simulink model "Pendulum"  (R2024b)
settings: Solver=FixedStepAuto  StartTime=0.0  StopTime=inf  RelTol=1e-3
libraries: slrealtimeethercatlib x13, simulink x2
settings Model: Creator=Wave User  LastModifiedBy=Wave User
settings SolverCC: ConcurrentTasks=on  PositivePriorityOrder=on
settings OptimizationCC: BlockReduction=off  OptimizeBlockIOStorage=off
settings DebuggingCC: TasksWithSamePriorityMsg=none
settings HardwareCC: ProdBitPerLong=64  ProdLongLongMode=on  ProdHWDeviceType=Intel->x86-64 (Linux 64)
settings RTWCC: Description=Speedgoat Real-Time Target Machine  SystemTargetFile=speedgoat.tlc  TemplateMakefile=slrealtime_default_tmf  Toolchain=Simulink Real-Time Toolchain  BuildConfiguration=Faster Runs  CodeExecutionProfiling=on  TargetLang=C++
settings SimulinkRealTimeTargetCC: InstructionSetFMA=off  LogToMDFFile=off

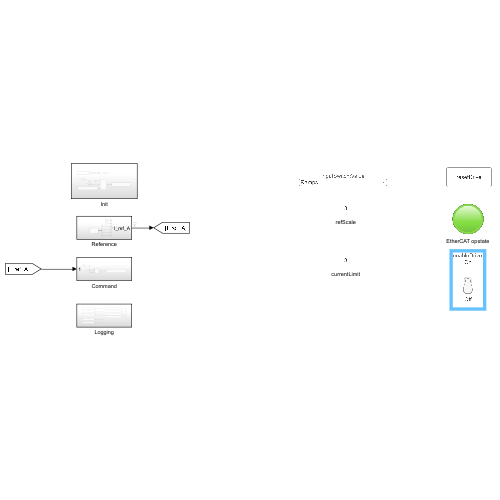
[thumbnail: Simulink's stored preview of the top-level diagram]
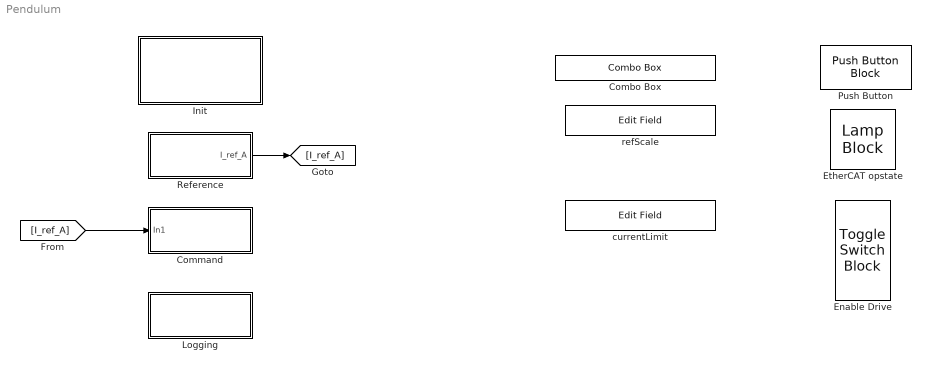
== system Pendulum ==
  Combo Box : ComboBox  SelectedLabel=Ramps
      settings: Values={{'Ramps', 'Sine', 'Chirp', 'BLWN', 'None'}, [2 3 4 5 1]}
  Command : Subsystem
  Enable Drive : ToggleSwitchBlock
      settings: Values={{'Off', 'On'}, [0 1]}
  EtherCAT opstate : LampBlock  LabelPosition=Hide
  Init : Subsystem
  Logging : Subsystem
  Push Button : PushButtonBlock  ButtonText=resetDrive  OffValue=0.000000
  Reference : Subsystem
  currentLimit : EditField  LabelPosition=Hide  ShowInitialText=on  Alignment=Center
  refScale : EditField  LabelPosition=Hide  ShowInitialText=on  Alignment=Center
  wires:
  Reference/1(I_ref_A) -> [I_ref_A]
  [I_ref_A] -> Command/1(In1)

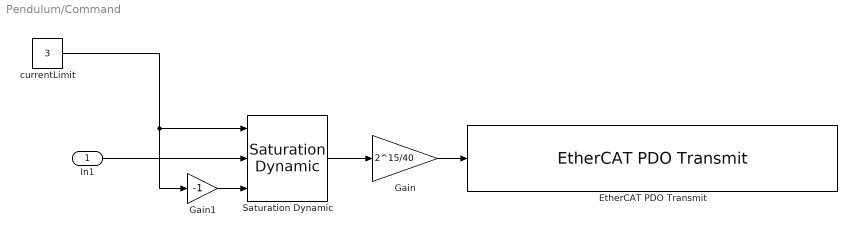
== system Pendulum/Command ==
  In1 : Inport
  EtherCAT PDO Transmit : slrealtimeethercatlib/EtherCAT PDO Transmit  Priority=3  sig_name=Drive 6 (AMC).Module 1 (Default).PDO data to Slave.Target Current  sig_offset=696  sig_type=int16  type_size=16  sig_dim=1  device_id=0  sample_time=0.001000
  Gain : Gain  Gain=2^15/40  OutDataTypeStr=int16
  Gain1 : Gain  Gain=-1
  Saturation Dynamic : simulink/Discontinuities/Saturation Dynamic  OutMin=[]  OutMax=[]  OutDataTypeStr=Inherit: Same as second input  OutDataType=fixdt(1, 16)  OutScaling=2^-10  DoSatur=off
  currentLimit : Constant  Value=3  OutDataTypeStr=Inherit: Inherit via back propagation
  wires:
  Saturation Dynamic/1 -> Gain/1
  Gain/1 -> EtherCAT PDO Transmit/1
  In1/1 -> Saturation Dynamic/2
  currentLimit/1 -> Gain1/1, Saturation Dynamic/1
  Gain1/1 -> Saturation Dynamic/3

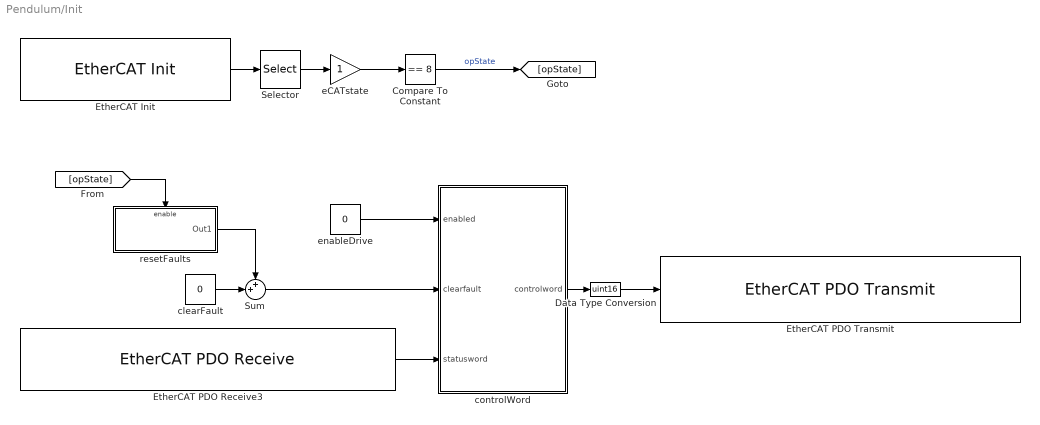
== system Pendulum/Init ==
  Compare To Constant : simulink/Logic and Bit Operations/Compare To Constant  relop===  const=8  OutDataTypeStr=boolean
  Data Type Conversion : DataTypeConversion  OutDataTypeStr=uint16  SaturateOnIntegerOverflow=off  RndMeth=Floor
  EtherCAT Init : slrealtimeethercatlib/EtherCAT Init  Priority=0  config_file=C:\Software\WEC-Bench\TwinCAT3\Pendulum2XML.xml  device_id=0  portnum=1  initstate=2  dctuning=0  enaDebug=0  logFile='c:\dbglog.txt'  sample_time=0.001000  DCMode=2
  EtherCAT PDO Receive3 : slrealtimeethercatlib/EtherCAT PDO Receive  Priority=2  sig_name=Drive 6 (AMC).Module 1 (Default).PDO data from Slave.Status Word  sig_offset=616  sig_type=uint16  type_size=16  sig_dim=1  device_id=0  sample_time=0.001000
  EtherCAT PDO Transmit : slrealtimeethercatlib/EtherCAT PDO Transmit  Priority=3  sig_name=Drive 6 (AMC).Module 1 (Default).PDO data to Slave.Control Word  sig_offset=616  sig_type=uint16  type_size=16  sig_dim=1  device_id=0  sample_time=0.001000
  Selector : Selector  InputPortWidth=6  IndexOptions=Index vector (dialog)  Indices=2  OutputSizes=1
  Sum : Sum  Inputs=++|
  clearFault : Constant  Value=0  OutDataTypeStr=Inherit: Inherit via back propagation
  controlWord : MATLAB Function  TreatAsAtomicUnit=on
  eCATstate : Gain  OutDataTypeStr=double
  enableDrive : Constant  Value=0
  resetFaults : Subsystem  TreatAsAtomicUnit=on
  wires:
  EtherCAT Init/1 -> Selector/1
  EtherCAT PDO Receive3/1 -> controlWord/3(statusword)
  eCATstate/1 -> Compare To Constant/1
  controlWord/1(controlword) -> Data Type Conversion/1
  Compare To Constant/1 -> [opState]  "opState"
  Selector/1 -> eCATstate/1
  enableDrive/1 -> controlWord/1(enabled)
  Sum/1 -> controlWord/2(clearfault)
  clearFault/1 -> Sum/2
  [opState] -> resetFaults/Enable
  resetFaults/1(Out1) -> Sum/1
  Data Type Conversion/1 -> EtherCAT PDO Transmit/1

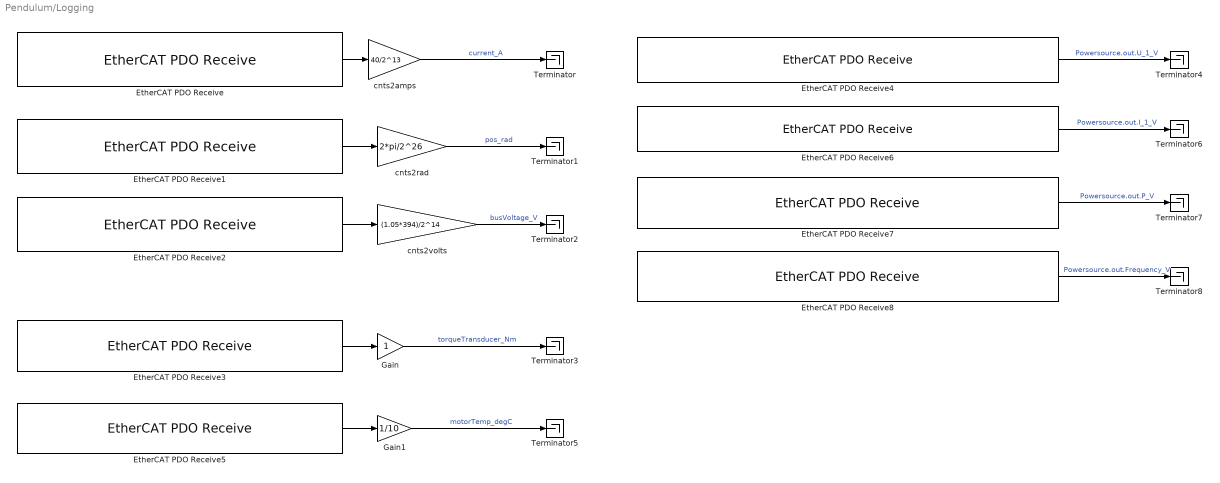
== system Pendulum/Logging ==
  EtherCAT PDO Receive : slrealtimeethercatlib/EtherCAT PDO Receive  Priority=2  sig_name=Drive 6 (AMC).Module 1 (Default).PDO data from Slave.Actual Current  sig_offset=696  sig_type=int16  type_size=16  sig_dim=1  device_id=0  sample_time=0.001000
  EtherCAT PDO Receive1 : slrealtimeethercatlib/EtherCAT PDO Receive  Priority=2  sig_name=Drive 6 (AMC).Module 1 (Default).PDO data from Slave.Actual position  sig_offset=632  sig_type=int32  type_size=32  sig_dim=1  device_id=0  sample_time=0.001000
  EtherCAT PDO Receive2 : slrealtimeethercatlib/EtherCAT PDO Receive  Priority=2  sig_name=Drive 6 (AMC).Module 1 (Default).PDO data from Slave.DC Bus Voltage  sig_offset=728  sig_type=int16  type_size=16  sig_dim=1  device_id=0  sample_time=0.001000
  EtherCAT PDO Receive3 : slrealtimeethercatlib/EtherCAT PDO Receive  Priority=2  sig_name=Term 4 (EL3356-0010).RMB Value (Real).Value (Real)  sig_offset=584  sig_type=single  type_size=32  sig_dim=1  device_id=0  sample_time=0.001000
  EtherCAT PDO Receive4 : slrealtimeethercatlib/EtherCAT PDO Receive  Priority=2  sig_name=Box 8 (GEN Series DAQ System).Powersource.out.U_1.Powersource.out.U_1_V  sig_offset=1336  sig_type=single  type_size=32  sig_dim=1  device_id=0  sample_time=0.001000
  EtherCAT PDO Receive5 : slrealtimeethercatlib/EtherCAT PDO Receive  Priority=2  sig_name=Term 5 (EL3201).RTD.Value  sig_offset=856  sig_type=int16  type_size=16  sig_dim=1  device_id=0  sample_time=0.001000
  EtherCAT PDO Receive6 : slrealtimeethercatlib/EtherCAT PDO Receive  Priority=2  sig_name=Box 8 (GEN Series DAQ System).Powersource.out.I_1.Powersource.out.I_1_V  sig_offset=1176  sig_type=single  type_size=32  sig_dim=1  device_id=0  sample_time=0.001000
  EtherCAT PDO Receive7 : slrealtimeethercatlib/EtherCAT PDO Receive  Priority=2  sig_name=Box 8 (GEN Series DAQ System).Powersource.out.P.Powersource.out.P_V  sig_offset=1616  sig_type=single  type_size=32  sig_dim=1  device_id=0  sample_time=0.001000
  EtherCAT PDO Receive8 : slrealtimeethercatlib/EtherCAT PDO Receive  Priority=2  sig_name=Box 8 (GEN Series DAQ System).Powersource.out.Frequency.Powersource.out.Frequency_V  sig_offset=1136  sig_type=single  type_size=32  sig_dim=1  device_id=0  sample_time=0.001000
  Gain : Gain  OutDataTypeStr=double
  Gain1 : Gain  Gain=1/10
  Terminator{,1..8} (9 alike) : Terminator
  cnts2amps : Gain  Gain=40/2^13  OutDataTypeStr=double
  cnts2rad : Gain  Gain=2*pi/2^26  OutDataTypeStr=double
  cnts2volts : Gain  Gain=(1.05*394)/2^14
  wires:
  EtherCAT PDO Receive/1 -> cnts2amps/1
  cnts2amps/1 -> Terminator/1  "current_A"
  EtherCAT PDO Receive1/1 -> cnts2rad/1
  cnts2rad/1 -> Terminator1/1  "pos_rad"
  EtherCAT PDO Receive2/1 -> cnts2volts/1
  cnts2volts/1 -> Terminator2/1  "busVoltage_V"
  EtherCAT PDO Receive3/1 -> Gain/1
  Gain/1 -> Terminator3/1  "torqueTransducer_Nm"
  EtherCAT PDO Receive4/1 -> Terminator4/1  "Powersource.out.U_1_V"
  EtherCAT PDO Receive5/1 -> Gain1/1
  Gain1/1 -> Terminator5/1  "motorTemp_degC"
  EtherCAT PDO Receive6/1 -> Terminator6/1  "Powersource.out.I_1_V"
  EtherCAT PDO Receive7/1 -> Terminator7/1  "Powersource.out.P_V"
  EtherCAT PDO Receive8/1 -> Terminator8/1  "Powersource.out.Frequency_V"

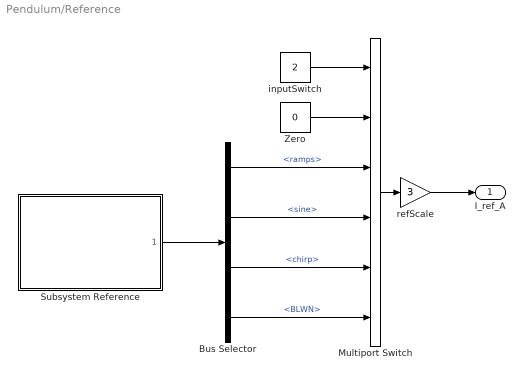
== system Pendulum/Reference ==
  Bus Selector : BusSelector  OutputSignals=ramps,sine,chirp,BLWN
  Multiport Switch : MultiPortSwitch  Inputs=5  SaturateOnIntegerOverflow=off  InputSameDT=off
  Subsystem Reference : Subsystem  ReferencedSubsystem=referenceSigs
  Zero : Constant  Value=0  OutDataTypeStr=Inherit: Inherit via back propagation
  inputSwitch : Constant  Value=2
  refScale : Gain  Gain=3
  I_ref_A : Outport
  wires:
  Subsystem Reference/1 -> Bus Selector/1
  Zero/1 -> Multiport Switch/2
  Bus Selector/1 -> Multiport Switch/3  "<ramps>"
  Bus Selector/2 -> Multiport Switch/4  "<sine>"
  Bus Selector/3 -> Multiport Switch/5  "<chirp>"
  Bus Selector/4 -> Multiport Switch/6  "<BLWN>"
  Multiport Switch/1 -> refScale/1
  inputSwitch/1 -> Multiport Switch/1
  refScale/1 -> I_ref_A/1

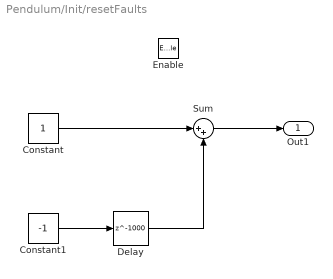
== system Pendulum/Init/resetFaults ==
  Enable : EnablePort
  Constant : Constant
  Constant1 : Constant  Value=-1
  Delay : Delay  DelayLength=1000
  Sum : Sum  Inputs=|++
  Out1 : Outport
  wires:
  Constant/1 -> Sum/1
  Constant1/1 -> Delay/1
  Delay/1 -> Sum/2
  Sum/1 -> Out1/1

== matlab function Pendulum/Init/controlWord ==
  data: enabled input; controlword output; clearfault input; statusword input
function controlword = fcn(enabled, clearfault, statusword)

bitstatus = bitget(statusword,1:16);

if ~clearfault
    if enabled
        if bitstatus(1) == 0 % Ready to switch on not ready
            controlword = 6; % command ready switch on
        elseif ~bitstatus(2) % switched not yet on
            controlword = 7; % command switch on
        elseif ~bitstatus(3) % operation not yet enabled
            controlword = 15; % command enable
        else
            controlword = 15; % maintain enabled state
        end
    else
        controlword = 4; % command disabled
    end
else
    controlword = 128; % command clear faults
end
